simulink model "saturn_thermal4"  (R2021a)
settings: Solver=ode23t  StartTime=0.0  StopTime=80000  MaxStep=1000  RelTol=1e-3
values from neighbouring files (symbols this model uses):
  Ab = L*l    [Data_ini_thermal_analysis4.m]    (also in Data_ini_thermal_analysis5.m)
  As = l*l    [Data_ini_thermal_analysis4.m]    (also in Data_ini_thermal_analysis5.m)
  D_st = 1224526    [Data_ini_thermal_analysis4.m]    (also in Data_ini_thermal_analysis5.m)
  ecc_sc = 0    [Data_ini_thermal_analysis4.m]    (also in Data_ini_thermal_analysis5.m)
  ecc_t = 0.0293    [Data_ini_thermal_analysis4.m]    (also in Data_ini_thermal_analysis5.m)
  incl_ax_s = deg2rad(26.73)    [Data_ini_thermal_analysis4.m]    (also in Data_ini_thermal_analysis5.m)
  incl_sc = deg2rad(90+45)    [Data_ini_thermal_analysis4.m]    (also in Data_ini_thermal_analysis5.m)
  incl_t = deg2rad(0.3485)    [Data_ini_thermal_analysis4.m]    (also in Data_ini_thermal_analysis5.m)
  mean_motion_sc = 2*pi/period_sc    [Data_ini_thermal_analysis4.m]    (also in Data_ini_thermal_analysis5.m)
  mean_motion_t = (2*pi)/period_t    (= 4.56068561416e-06)    [Data_ini_thermal_analysis4.m]    (also in Data_ini_thermal_analysis5.m)
  mean_r_s = 1.427*10^9    (= 1427000000)    [Data_ini_thermal_analysis4.m]    (also in Data_ini_thermal_analysis5.m)
  mu_s = 37931187    [Data_ini_thermal_analysis4.m]    (also in Data_ini_thermal_analysis5.m)
  mu_t = 8971.15    [Data_ini_thermal_analysis4.m]    (also in Data_ini_thermal_analysis5.m)
  period_s = 29.45*365*24*3600    (= 928735200)    [Data_ini_thermal_analysis4.m]    (also in Data_ini_thermal_analysis5.m)
  period_t = 15.945421*24*3600    (= 1377684.3744)    [Data_ini_thermal_analysis4.m]    (also in Data_ini_thermal_analysis5.m)
  R_s = diam_s/2    (= 60268)    [Data_ini_thermal_analysis4.m]    (also in Data_ini_thermal_analysis5.m)
  R_t = 2576    [Data_ini_thermal_analysis4.m]    (also in Data_ini_thermal_analysis5.m)
  semajax_sc = 1500+R_t    (= 4076)    [Data_ini_thermal_analysis4.m]    (also in Data_ini_thermal_analysis5.m)
  semajax_t = 1221830    [Data_ini_thermal_analysis4.m]    (also in Data_ini_thermal_analysis5.m)
libraries: fl_lib x283, nesl_utility x27
(part 2 of 3)

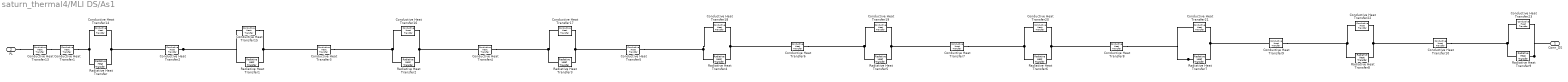
== system saturn_thermal4/MLI DS/As1 ==
  Conductive Heat Transfer{1..10} (10 alike) : fl_lib/Thermal/Thermal Elements/Conductive Heat Transfer  area=As m^2  thickness=s_kap m  th_cond=k_kap W/(m*K)  T_specify=off  T_priority=None  T=0 K  T_nominal_specify=off  T_nominal_unit=K  T_nominal_value=1  Q_specify=off  Q_priority=None  Q=0 W  Q_nominal_specify=off  Q_nominal_unit=W  Q_nominal_value=1
  Conductive Heat Transfer13 : fl_lib/Thermal/Thermal Elements/Conductive Heat Transfer  area=As m^2  thickness=s_al m  th_cond=k_al W/(m*K)  T_specify=off  T_priority=None  T=0 K  T_nominal_specify=off  T_nominal_unit=K  T_nominal_value=1  Q_specify=off  Q_priority=None  Q=0 W  Q_nominal_specify=off  Q_nominal_unit=W  Q_nominal_value=1
  Conductive Heat Transfer{14..23} (10 alike) : fl_lib/Thermal/Thermal Elements/Conductive Heat Transfer  area=A_net_new m^2  thickness=s_tfe_out m  th_cond=k_tfe W/(m*K)  T_specify=off  T_priority=None  T=0 K  T_nominal_specify=off  T_nominal_unit=K  T_nominal_value=1  Q_specify=off  Q_priority=None  Q=0 W  Q_nominal_specify=off  Q_nominal_unit=W  Q_nominal_value=1
  Radiative Heat Transfer{,1..9} (10 alike) : fl_lib/Thermal/Thermal Elements/Radiative Heat Transfer  area=A_empty m^2  rad_tr_coeff=Gr_kap_mli W/(m^2*K^4)  T_specify=off  T_priority=None  T=0 K  T_nominal_specify=off  T_nominal_unit=K  T_nominal_value=1  Q_specify=off  Q_priority=None  Q=0 W  Q_nominal_specify=off  Q_nominal_unit=W  Q_nominal_value=1
      settings: SourceProductBaseCode=SS  InternalSimscapePortConfiguration="{\"Bottom\":[],\"Left\":[{\"id\":\"A\",\"label\":\"A\",\"type\":\"foundation.thermal.thermal\"}],\"Right\":[{\"id\":\"B\",\"label\":\"B\",\"type\":\"foundation.thermal.thermal\"}],\"Top\":[]}"
  Conn_DS : PMIOPort  Side=Right
  PL : PMIOPort  Port=2  Side=Left
  connections:
  Radiative Heat Transfer/LConn1 -- Conductive Heat Transfer14/LConn1 -- Conductive Heat Transfer1/RConn1
  PL/RConn1 -- Conductive Heat Transfer13/LConn1
  Conductive Heat Transfer10/LConn1 -- Conductive Heat Transfer22/RConn1 -- Radiative Heat Transfer8/RConn1
  Conductive Heat Transfer9/RConn1 -- Conductive Heat Transfer22/LConn1 -- Radiative Heat Transfer8/LConn1
  Conductive Heat Transfer2/RConn1 -- Radiative Heat Transfer1/LConn1 -- Conductive Heat Transfer15/LConn1
  Radiative Heat Transfer9/RConn1 -- Conn_DS/RConn1 -- Conductive Heat Transfer23/RConn1
  Conductive Heat Transfer3/LConn1 -- Conductive Heat Transfer15/RConn1 -- Radiative Heat Transfer1/RConn1
  Conductive Heat Transfer4/LConn1 -- Conductive Heat Transfer16/RConn1 -- Radiative Heat Transfer2/RConn1
  Conductive Heat Transfer3/RConn1 -- Conductive Heat Transfer16/LConn1 -- Radiative Heat Transfer2/LConn1
  Conductive Heat Transfer2/LConn1 -- Radiative Heat Transfer/RConn1 -- Conductive Heat Transfer14/RConn1
  Conductive Heat Transfer10/RConn1 -- Conductive Heat Transfer23/LConn1 -- Radiative Heat Transfer9/LConn1
  Conductive Heat Transfer5/LConn1 -- Conductive Heat Transfer17/RConn1 -- Radiative Heat Transfer3/RConn1
  Conductive Heat Transfer6/LConn1 -- Conductive Heat Transfer18/RConn1 -- Radiative Heat Transfer4/RConn1
  Conductive Heat Transfer9/LConn1 -- Conductive Heat Transfer21/RConn1 -- Radiative Heat Transfer7/RConn1
  Conductive Heat Transfer7/RConn1 -- Conductive Heat Transfer20/LConn1 -- Radiative Heat Transfer6/LConn1
  Conductive Heat Transfer5/RConn1 -- Conductive Heat Transfer18/LConn1 -- Radiative Heat Transfer4/LConn1
  Conductive Heat Transfer13/RConn1 -- Conductive Heat Transfer1/LConn1
  Conductive Heat Transfer7/LConn1 -- Conductive Heat Transfer19/RConn1 -- Radiative Heat Transfer5/RConn1
  Conductive Heat Transfer4/RConn1 -- Radiative Heat Transfer3/LConn1 -- Conductive Heat Transfer17/LConn1
  Radiative Heat Transfer7/LConn1 -- Conductive Heat Transfer8/RConn1 -- Conductive Heat Transfer21/LConn1
  Conductive Heat Transfer8/LConn1 -- Conductive Heat Transfer20/RConn1 -- Radiative Heat Transfer6/RConn1
  Conductive Heat Transfer6/RConn1 -- Conductive Heat Transfer19/LConn1 -- Radiative Heat Transfer5/LConn1

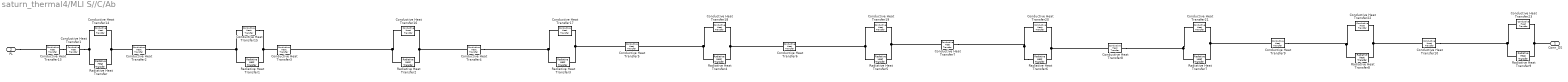
== system saturn_thermal4/MLI S//C/Ab ==
  Conductive Heat Transfer{1..10} (10 alike) : fl_lib/Thermal/Thermal Elements/Conductive Heat Transfer  area=Ab m^2  thickness=s_kap m  th_cond=k_kap W/(m*K)  T_specify=off  T_priority=None  T=0 K  T_nominal_specify=off  T_nominal_unit=K  T_nominal_value=1  Q_specify=off  Q_priority=None  Q=0 W  Q_nominal_specify=off  Q_nominal_unit=W  Q_nominal_value=1
  Conductive Heat Transfer13 : fl_lib/Thermal/Thermal Elements/Conductive Heat Transfer  area=Ab m^2  thickness=s_al m  th_cond=k_al W/(m*K)  T_specify=off  T_priority=None  T=0 K  T_nominal_specify=off  T_nominal_unit=K  T_nominal_value=1  Q_specify=off  Q_priority=None  Q=0 W  Q_nominal_specify=off  Q_nominal_unit=W  Q_nominal_value=1
  Conductive Heat Transfer{14..23} (10 alike) : fl_lib/Thermal/Thermal Elements/Conductive Heat Transfer  area=A_net_new_b m^2  thickness=s_tfe_out m  th_cond=k_tfe W/(m*K)  T_specify=off  T_priority=None  T=0 K  T_nominal_specify=off  T_nominal_unit=K  T_nominal_value=1  Q_specify=off  Q_priority=None  Q=0 W  Q_nominal_specify=off  Q_nominal_unit=W  Q_nominal_value=1
  Radiative Heat Transfer{,1..9} (10 alike) : fl_lib/Thermal/Thermal Elements/Radiative Heat Transfer  area=A_empty_b m^2  rad_tr_coeff=Gr_kap_mli W/(m^2*K^4)  T_specify=off  T_priority=None  T=0 K  T_nominal_specify=off  T_nominal_unit=K  T_nominal_value=1  Q_specify=off  Q_priority=None  Q=0 W  Q_nominal_specify=off  Q_nominal_unit=W  Q_nominal_value=1
      settings: SourceProductBaseCode=SS  InternalSimscapePortConfiguration="{\"Bottom\":[],\"Left\":[{\"id\":\"A\",\"label\":\"A\",\"type\":\"foundation.thermal.thermal\"}],\"Right\":[{\"id\":\"B\",\"label\":\"B\",\"type\":\"foundation.thermal.thermal\"}],\"Top\":[]}"
  Conn_DS : PMIOPort  Side=Right
  PL : PMIOPort  Port=2  Side=Left
  connections:
  Conductive Heat Transfer13/RConn1 -- Conductive Heat Transfer1/LConn1
  PL/RConn1 -- Conductive Heat Transfer13/LConn1
  Conductive Heat Transfer10/LConn1 -- Conductive Heat Transfer22/RConn1 -- Radiative Heat Transfer8/RConn1
  Conductive Heat Transfer9/RConn1 -- Conductive Heat Transfer22/LConn1 -- Radiative Heat Transfer8/LConn1
  Conductive Heat Transfer2/RConn1 -- Radiative Heat Transfer1/LConn1 -- Conductive Heat Transfer15/LConn1
  Conn_DS/RConn1 -- Conductive Heat Transfer23/RConn1 -- Radiative Heat Transfer9/RConn1
  Radiative Heat Transfer1/RConn1 -- Conductive Heat Transfer15/RConn1 -- Conductive Heat Transfer3/LConn1
  Conductive Heat Transfer4/LConn1 -- Conductive Heat Transfer16/RConn1 -- Radiative Heat Transfer2/RConn1
  Conductive Heat Transfer3/RConn1 -- Conductive Heat Transfer16/LConn1 -- Radiative Heat Transfer2/LConn1
  Conductive Heat Transfer2/LConn1 -- Conductive Heat Transfer14/RConn1 -- Radiative Heat Transfer/RConn1
  Conductive Heat Transfer10/RConn1 -- Conductive Heat Transfer23/LConn1 -- Radiative Heat Transfer9/LConn1
  Radiative Heat Transfer3/RConn1 -- Conductive Heat Transfer17/RConn1 -- Conductive Heat Transfer5/LConn1
  Conductive Heat Transfer6/LConn1 -- Radiative Heat Transfer4/RConn1 -- Conductive Heat Transfer18/RConn1
  Radiative Heat Transfer7/RConn1 -- Conductive Heat Transfer21/RConn1 -- Conductive Heat Transfer9/LConn1
  Radiative Heat Transfer6/LConn1 -- Conductive Heat Transfer20/LConn1 -- Conductive Heat Transfer7/RConn1
  Conductive Heat Transfer5/RConn1 -- Conductive Heat Transfer18/LConn1 -- Radiative Heat Transfer4/LConn1
  Conductive Heat Transfer14/LConn1 -- Conductive Heat Transfer1/RConn1 -- Radiative Heat Transfer/LConn1
  Conductive Heat Transfer7/LConn1 -- Conductive Heat Transfer19/RConn1 -- Radiative Heat Transfer5/RConn1
  Conductive Heat Transfer4/RConn1 -- Radiative Heat Transfer3/LConn1 -- Conductive Heat Transfer17/LConn1
  Conductive Heat Transfer8/RConn1 -- Radiative Heat Transfer7/LConn1 -- Conductive Heat Transfer21/LConn1
  Conductive Heat Transfer8/LConn1 -- Radiative Heat Transfer6/RConn1 -- Conductive Heat Transfer20/RConn1
  Conductive Heat Transfer6/RConn1 -- Radiative Heat Transfer5/LConn1 -- Conductive Heat Transfer19/LConn1

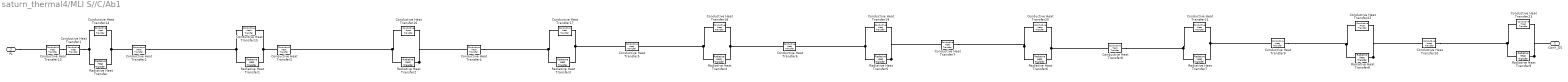
== system saturn_thermal4/MLI S//C/Ab1 ==
  Conductive Heat Transfer{1..10} (10 alike) : fl_lib/Thermal/Thermal Elements/Conductive Heat Transfer  area=Ab m^2  thickness=s_kap m  th_cond=k_kap W/(m*K)  T_specify=off  T_priority=None  T=0 K  T_nominal_specify=off  T_nominal_unit=K  T_nominal_value=1  Q_specify=off  Q_priority=None  Q=0 W  Q_nominal_specify=off  Q_nominal_unit=W  Q_nominal_value=1
  Conductive Heat Transfer13 : fl_lib/Thermal/Thermal Elements/Conductive Heat Transfer  area=Ab m^2  thickness=s_al m  th_cond=k_al W/(m*K)  T_specify=off  T_priority=None  T=0 K  T_nominal_specify=off  T_nominal_unit=K  T_nominal_value=1  Q_specify=off  Q_priority=None  Q=0 W  Q_nominal_specify=off  Q_nominal_unit=W  Q_nominal_value=1
  Conductive Heat Transfer{14..23} (10 alike) : fl_lib/Thermal/Thermal Elements/Conductive Heat Transfer  area=A_net_new_b m^2  thickness=s_tfe_out m  th_cond=k_tfe W/(m*K)  T_specify=off  T_priority=None  T=0 K  T_nominal_specify=off  T_nominal_unit=K  T_nominal_value=1  Q_specify=off  Q_priority=None  Q=0 W  Q_nominal_specify=off  Q_nominal_unit=W  Q_nominal_value=1
  Radiative Heat Transfer{,1..9} (10 alike) : fl_lib/Thermal/Thermal Elements/Radiative Heat Transfer  area=A_empty_b m^2  rad_tr_coeff=Gr_kap_mli W/(m^2*K^4)  T_specify=off  T_priority=None  T=0 K  T_nominal_specify=off  T_nominal_unit=K  T_nominal_value=1  Q_specify=off  Q_priority=None  Q=0 W  Q_nominal_specify=off  Q_nominal_unit=W  Q_nominal_value=1
      settings: SourceProductBaseCode=SS  InternalSimscapePortConfiguration="{\"Bottom\":[],\"Left\":[{\"id\":\"A\",\"label\":\"A\",\"type\":\"foundation.thermal.thermal\"}],\"Right\":[{\"id\":\"B\",\"label\":\"B\",\"type\":\"foundation.thermal.thermal\"}],\"Top\":[]}"
  Conn_DS : PMIOPort  Side=Right
  PL : PMIOPort  Port=2  Side=Left
  connections:
  Conductive Heat Transfer19/LConn1 -- Radiative Heat Transfer5/LConn1 -- Conductive Heat Transfer6/RConn1
  Conductive Heat Transfer20/RConn1 -- Radiative Heat Transfer6/RConn1 -- Conductive Heat Transfer8/LConn1
  Conductive Heat Transfer21/LConn1 -- Radiative Heat Transfer7/LConn1 -- Conductive Heat Transfer8/RConn1
  Conductive Heat Transfer17/LConn1 -- Radiative Heat Transfer3/LConn1 -- Conductive Heat Transfer4/RConn1
  Radiative Heat Transfer5/RConn1 -- Conductive Heat Transfer19/RConn1 -- Conductive Heat Transfer7/LConn1
  Radiative Heat Transfer/LConn1 -- Conductive Heat Transfer1/RConn1 -- Conductive Heat Transfer14/LConn1
  Radiative Heat Transfer4/LConn1 -- Conductive Heat Transfer18/LConn1 -- Conductive Heat Transfer5/RConn1
  Conductive Heat Transfer7/RConn1 -- Conductive Heat Transfer20/LConn1 -- Radiative Heat Transfer6/LConn1
  Conductive Heat Transfer9/LConn1 -- Conductive Heat Transfer21/RConn1 -- Radiative Heat Transfer7/RConn1
  Conductive Heat Transfer18/RConn1 -- Radiative Heat Transfer4/RConn1 -- Conductive Heat Transfer6/LConn1
  Conductive Heat Transfer5/LConn1 -- Conductive Heat Transfer17/RConn1 -- Radiative Heat Transfer3/RConn1
  Radiative Heat Transfer9/LConn1 -- Conductive Heat Transfer23/LConn1 -- Conductive Heat Transfer10/RConn1
  Radiative Heat Transfer/RConn1 -- Conductive Heat Transfer14/RConn1 -- Conductive Heat Transfer2/LConn1
  Radiative Heat Transfer2/LConn1 -- Conductive Heat Transfer16/LConn1 -- Conductive Heat Transfer3/RConn1
  Radiative Heat Transfer2/RConn1 -- Conductive Heat Transfer16/RConn1 -- Conductive Heat Transfer4/LConn1
  Conductive Heat Transfer3/LConn1 -- Conductive Heat Transfer15/RConn1 -- Radiative Heat Transfer1/RConn1
  Radiative Heat Transfer9/RConn1 -- Conductive Heat Transfer23/RConn1 -- Conn_DS/RConn1
  Conductive Heat Transfer15/LConn1 -- Radiative Heat Transfer1/LConn1 -- Conductive Heat Transfer2/RConn1
  Radiative Heat Transfer8/LConn1 -- Conductive Heat Transfer22/LConn1 -- Conductive Heat Transfer9/RConn1
  Radiative Heat Transfer8/RConn1 -- Conductive Heat Transfer22/RConn1 -- Conductive Heat Transfer10/LConn1
  PL/RConn1 -- Conductive Heat Transfer13/LConn1
  Conductive Heat Transfer13/RConn1 -- Conductive Heat Transfer1/LConn1

== system saturn_thermal4/active heat control box/Subsystem ==
  signal : Inport
  reference : Inport  Port=2
  on case : Inport  Port=3
  off case : Inport  Port=4
  Controlled Heat Flow Rate Source : fl_lib/Thermal/Thermal Sources/Controlled Heat Flow Rate Source
  Data Type Conversion : DataTypeConversion  OutDataTypeStr=double
  Relational Operator : RelationalOperator  Operator=<=  OutDataTypeStr=boolean  RndMeth=Simplest
  Simulink-PS Converter : nesl_utility/Simulink-PS Converter  PhysicalDomain=network_engine_domain  SubClassName=ps_input  LeftPortType=input  RightPortType=output  PseudoPeriodic=off  Frequencies=[]  NoiseDistribution=none  NoiseParameters=[]  Unit=1  AffineConversion=off  FilteringAndDerivatives=provide  SimscapeFilterOrder=1  InputFilterTimeConstant=0.001  UdotUserProvided=0
      settings: SourceProductBaseCode=PW,SS
  Switch : Switch  Criteria=u2 > Threshold
  Thermal Reference1 : fl_lib/Thermal/Thermal Elements/Thermal Reference
  heat block : PMIOPort  Side=Right
  Output : Outport
  wires:
  Data Type Conversion/1 -> Simulink-PS Converter/1
  signal/1 -> Relational Operator/1
  off case/1 -> Switch/3
  Relational Operator/1 -> Output/1, Switch/2
  Switch/1 -> Data Type Conversion/1
  reference/1 -> Relational Operator/2
  on case/1 -> Switch/1
  connections:
  Thermal Reference1/LConn1 -- Controlled Heat Flow Rate Source/RConn2
  Controlled Heat Flow Rate Source/LConn1 -- heat block/RConn1
  Simulink-PS Converter/RConn1 -- Controlled Heat Flow Rate Source/RConn1

== system saturn_thermal4/active heat control box/Subsystem1 ==
  signal : Inport
  reference : Inport  Port=2
  off case : Inport  Port=3
  Conductive Heat Transfer1 : fl_lib/Thermal/Thermal Elements/Conductive Heat Transfer  area=As m^2  thickness=0.3 m  th_cond=k_al W/(m*K)  T_specify=off  T_priority=None  T=0 K  T_nominal_specify=off  T_nominal_unit=K  T_nominal_value=1  Q_specify=off  Q_priority=None  Q=0 W  Q_nominal_specify=off  Q_nominal_unit=W  Q_nominal_value=1
  Controlled Temperature Source : fl_lib/Thermal/Thermal Sources/Controlled Temperature Source
  Data Type Conversion : DataTypeConversion  OutDataTypeStr=double
  Deep space1 : fl_lib/Thermal/Thermal Sources/Temperature Source  temperature=T_ds K
  PS-Simulink Converter : nesl_utility/PS-Simulink Converter  PhysicalDomain=network_engine_domain  SubClassName=ps_output  LeftPortType=input  RightPortType=output  PseudoPeriodic=off  Frequencies=[]  Unit=inherit  AffineConversion=off
      settings: SourceProductBaseCode=PW,SS
  Radiative Heat Transfer3 : fl_lib/Thermal/Thermal Elements/Radiative Heat Transfer  area=5*As m^2  rad_tr_coeff=Gr_al W/(m^2*K^4)  T_specify=off  T_priority=None  T=0 K  T_nominal_specify=off  T_nominal_unit=K  T_nominal_value=1  Q_specify=off  Q_priority=None  Q=0 W  Q_nominal_specify=off  Q_nominal_unit=W  Q_nominal_value=1
      settings: SourceProductBaseCode=SS  InternalSimscapePortConfiguration="{\"Bottom\":[],\"Left\":[{\"id\":\"A\",\"label\":\"A\",\"type\":\"foundation.thermal.thermal\"}],\"Right\":[{\"id\":\"B\",\"label\":\"B\",\"type\":\"foundation.thermal.thermal\"}],\"Top\":[]}"
  Radiator : fl_lib/Thermal/Thermal Elements/Thermal Mass  mass=m_rad kg  sp_heat=cp_al J/kg/K  T_specify=on  T_priority=High  T=3 K  T_nominal_specify=off  T_nominal_unit=K  T_nominal_value=1  Q_specify=off  Q_priority=None  Q=0 W  Q_nominal_specify=off  Q_nominal_unit=W  Q_nominal_value=1
  Relational Operator : RelationalOperator  OutDataTypeStr=boolean  RndMeth=Simplest
  Simulink-PS Converter : nesl_utility/Simulink-PS Converter  PhysicalDomain=network_engine_domain  SubClassName=ps_input  LeftPortType=input  RightPortType=output  PseudoPeriodic=off  Frequencies=[]  NoiseDistribution=none  NoiseParameters=[]  Unit=1  AffineConversion=off  FilteringAndDerivatives=provide  SimscapeFilterOrder=1  InputFilterTimeConstant=0.001  UdotUserProvided=0
      settings: SourceProductBaseCode=PW,SS
  Solver Configuration : nesl_utility/Solver Configuration  PhysicalDomain=network_engine_domain  SubClassName=solver  LeftPortType=input  RightPortType=generic  Tones=[]  Harmonics=[]  SimulateNoise=off  Profile=off  UseLocalSampling=off  EnableSwitchedLinearOptims=on  FrequencyDomain=off  UseCCode=off  RelTol=0.001  AbsTol=1e-06  MinStep=1e-09  ToWorkspace=off  RevertToSquareIcSolve=off  NumHomotopyIterations=100  PhasorMode=off  PhasorModeNumHarmonics=1  DoDC=off  ResidualTolerance=1e-09  UseLocalSolver=off  LocalSolverChoice=NE_BACKWARD_EULER_ADVANCER  LocalSolverSampleTime=0.001  DoFixedCost=off  MaxNonlinIter=3  MaxModeIter=2  ComputeImpulses=off  ImpulseIterations=2  LinearAlgebra=auto  EquationFormulation=NE_TIME_EF  DelaysMemoryBudget=1024  AutomaticFiltering=on  FilteringTimeConstant=0.001  PartitionStorageMethod=AS_NEEDED  PartitionMemoryBudget=1024  PartitionMethod=ROBUST
      settings: SourceProductBaseCode=PW,SS
  Switch : Switch  Criteria=u2 > Threshold
  Temperature Sensor : fl_lib/Thermal/Thermal Sensors/Temperature Sensor
  Thermal Reference1 : fl_lib/Thermal/Thermal Elements/Thermal Reference
  Thermal Reference2 : fl_lib/Thermal/Thermal Elements/Thermal Reference
  heat block : PMIOPort  Side=Left
  Output : Outport
  wires:
  reference/1 -> Relational Operator/2
  Switch/1 -> Data Type Conversion/1
  Relational Operator/1 -> Output/1, Switch/2
  off case/1 -> Switch/3
  signal/1 -> Relational Operator/1
  Data Type Conversion/1 -> Simulink-PS Converter/1
  PS-Simulink Converter/1 -> Switch/1
  connections:
  Simulink-PS Converter/RConn1 -- Controlled Temperature Source/RConn1
  Solver Configuration/RConn1 -- Thermal Reference1/LConn1 -- Controlled Temperature Source/RConn2
  heat block/RConn1 -- Temperature Sensor/LConn1
  Temperature Sensor/RConn2 -- PS-Simulink Converter/LConn1
  Temperature Sensor/RConn1 -- Thermal Reference2/LConn1
  Conductive Heat Transfer1/RConn1 -- Radiative Heat Transfer3/LConn1 -- Radiator/LConn1
  Controlled Temperature Source/LConn1 -- Conductive Heat Transfer1/LConn1
  Radiative Heat Transfer3/RConn1 -- Deep space1/LConn1

== system saturn_thermal4/active heat control ref + antenna/Subsystem ==
  signal : Inport
  reference : Inport  Port=2
  on case : Inport  Port=3
  off case : Inport  Port=4
  Controlled Heat Flow Rate Source : fl_lib/Thermal/Thermal Sources/Controlled Heat Flow Rate Source
  Data Type Conversion : DataTypeConversion  OutDataTypeStr=double
  Relational Operator : RelationalOperator  Operator=<=  OutDataTypeStr=boolean  RndMeth=Simplest
  Simulink-PS Converter : nesl_utility/Simulink-PS Converter  PhysicalDomain=network_engine_domain  SubClassName=ps_input  LeftPortType=input  RightPortType=output  PseudoPeriodic=off  Frequencies=[]  NoiseDistribution=none  NoiseParameters=[]  Unit=1  AffineConversion=off  FilteringAndDerivatives=provide  SimscapeFilterOrder=1  InputFilterTimeConstant=0.001  UdotUserProvided=0
      settings: SourceProductBaseCode=PW,SS
  Switch : Switch  Criteria=u2 > Threshold
  Thermal Reference1 : fl_lib/Thermal/Thermal Elements/Thermal Reference
  heat block : PMIOPort  Side=Right
  Output : Outport
  wires:
  Data Type Conversion/1 -> Simulink-PS Converter/1
  signal/1 -> Relational Operator/1
  off case/1 -> Switch/3
  Relational Operator/1 -> Output/1, Switch/2
  Switch/1 -> Data Type Conversion/1
  reference/1 -> Relational Operator/2
  on case/1 -> Switch/1
  connections:
  Thermal Reference1/LConn1 -- Controlled Heat Flow Rate Source/RConn2
  Controlled Heat Flow Rate Source/LConn1 -- heat block/RConn1
  Simulink-PS Converter/RConn1 -- Controlled Heat Flow Rate Source/RConn1

== system saturn_thermal4/active heat control ref + antenna/Subsystem1 ==
  signal : Inport
  reference : Inport  Port=2
  off case : Inport  Port=3
  Conductive Heat Transfer1 : fl_lib/Thermal/Thermal Elements/Conductive Heat Transfer  area=As m^2  thickness=0.3 m  th_cond=k_al W/(m*K)  T_specify=off  T_priority=None  T=0 K  T_nominal_specify=off  T_nominal_unit=K  T_nominal_value=1  Q_specify=off  Q_priority=None  Q=0 W  Q_nominal_specify=off  Q_nominal_unit=W  Q_nominal_value=1
  Controlled Temperature Source : fl_lib/Thermal/Thermal Sources/Controlled Temperature Source
  Data Type Conversion : DataTypeConversion  OutDataTypeStr=double
  Deep space1 : fl_lib/Thermal/Thermal Sources/Temperature Source  temperature=T_ds K
  PS-Simulink Converter : nesl_utility/PS-Simulink Converter  PhysicalDomain=network_engine_domain  SubClassName=ps_output  LeftPortType=input  RightPortType=output  PseudoPeriodic=off  Frequencies=[]  Unit=inherit  AffineConversion=off
      settings: SourceProductBaseCode=PW,SS
  Radiative Heat Transfer3 : fl_lib/Thermal/Thermal Elements/Radiative Heat Transfer  area=5*As m^2  rad_tr_coeff=Gr_al W/(m^2*K^4)  T_specify=off  T_priority=None  T=0 K  T_nominal_specify=off  T_nominal_unit=K  T_nominal_value=1  Q_specify=off  Q_priority=None  Q=0 W  Q_nominal_specify=off  Q_nominal_unit=W  Q_nominal_value=1
      settings: SourceProductBaseCode=SS  InternalSimscapePortConfiguration="{\"Bottom\":[],\"Left\":[{\"id\":\"A\",\"label\":\"A\",\"type\":\"foundation.thermal.thermal\"}],\"Right\":[{\"id\":\"B\",\"label\":\"B\",\"type\":\"foundation.thermal.thermal\"}],\"Top\":[]}"
  Radiator : fl_lib/Thermal/Thermal Elements/Thermal Mass  mass=m_rad kg  sp_heat=cp_al J/kg/K  T_specify=on  T_priority=High  T=3 K  T_nominal_specify=off  T_nominal_unit=K  T_nominal_value=1  Q_specify=off  Q_priority=None  Q=0 W  Q_nominal_specify=off  Q_nominal_unit=W  Q_nominal_value=1
  Relational Operator : RelationalOperator  OutDataTypeStr=boolean  RndMeth=Simplest
  Simulink-PS Converter : nesl_utility/Simulink-PS Converter  PhysicalDomain=network_engine_domain  SubClassName=ps_input  LeftPortType=input  RightPortType=output  PseudoPeriodic=off  Frequencies=[]  NoiseDistribution=none  NoiseParameters=[]  Unit=1  AffineConversion=off  FilteringAndDerivatives=provide  SimscapeFilterOrder=1  InputFilterTimeConstant=0.001  UdotUserProvided=0
      settings: SourceProductBaseCode=PW,SS
  Solver Configuration : nesl_utility/Solver Configuration  PhysicalDomain=network_engine_domain  SubClassName=solver  LeftPortType=input  RightPortType=generic  Tones=[]  Harmonics=[]  SimulateNoise=off  Profile=off  UseLocalSampling=off  EnableSwitchedLinearOptims=on  FrequencyDomain=off  UseCCode=off  RelTol=0.001  AbsTol=1e-06  MinStep=1e-09  ToWorkspace=off  RevertToSquareIcSolve=off  NumHomotopyIterations=100  PhasorMode=off  PhasorModeNumHarmonics=1  DoDC=off  ResidualTolerance=1e-09  UseLocalSolver=off  LocalSolverChoice=NE_BACKWARD_EULER_ADVANCER  LocalSolverSampleTime=0.001  DoFixedCost=off  MaxNonlinIter=3  MaxModeIter=2  ComputeImpulses=off  ImpulseIterations=2  LinearAlgebra=auto  EquationFormulation=NE_TIME_EF  DelaysMemoryBudget=1024  AutomaticFiltering=on  FilteringTimeConstant=0.001  PartitionStorageMethod=AS_NEEDED  PartitionMemoryBudget=1024  PartitionMethod=ROBUST
      settings: SourceProductBaseCode=PW,SS
  Switch : Switch  Criteria=u2 > Threshold
  Temperature Sensor : fl_lib/Thermal/Thermal Sensors/Temperature Sensor
  Thermal Reference1 : fl_lib/Thermal/Thermal Elements/Thermal Reference
  Thermal Reference2 : fl_lib/Thermal/Thermal Elements/Thermal Reference
  heat block : PMIOPort  Side=Left
  Output : Outport
  wires:
  reference/1 -> Relational Operator/2
  Switch/1 -> Data Type Conversion/1
  Relational Operator/1 -> Output/1, Switch/2
  off case/1 -> Switch/3
  signal/1 -> Relational Operator/1
  Data Type Conversion/1 -> Simulink-PS Converter/1
  PS-Simulink Converter/1 -> Switch/1
  connections:
  Simulink-PS Converter/RConn1 -- Controlled Temperature Source/RConn1
  Solver Configuration/RConn1 -- Thermal Reference1/LConn1 -- Controlled Temperature Source/RConn2
  heat block/RConn1 -- Temperature Sensor/LConn1
  Temperature Sensor/RConn2 -- PS-Simulink Converter/LConn1
  Temperature Sensor/RConn1 -- Thermal Reference2/LConn1
  Conductive Heat Transfer1/RConn1 -- Radiative Heat Transfer3/LConn1 -- Radiator/LConn1
  Controlled Temperature Source/LConn1 -- Conductive Heat Transfer1/LConn1
  Radiative Heat Transfer3/RConn1 -- Deep space1/LConn1

== system saturn_thermal4/active heat control ref + antenna1/Subsystem ==
  signal : Inport
  reference : Inport  Port=2
  on case : Inport  Port=3
  off case : Inport  Port=4
  Controlled Heat Flow Rate Source : fl_lib/Thermal/Thermal Sources/Controlled Heat Flow Rate Source
  Data Type Conversion : DataTypeConversion  OutDataTypeStr=double
  Relational Operator : RelationalOperator  Operator=<=  OutDataTypeStr=boolean  RndMeth=Simplest
  Simulink-PS Converter : nesl_utility/Simulink-PS Converter  PhysicalDomain=network_engine_domain  SubClassName=ps_input  LeftPortType=input  RightPortType=output  PseudoPeriodic=off  Frequencies=[]  NoiseDistribution=none  NoiseParameters=[]  Unit=1  AffineConversion=off  FilteringAndDerivatives=provide  SimscapeFilterOrder=1  InputFilterTimeConstant=0.001  UdotUserProvided=0
      settings: SourceProductBaseCode=PW,SS
  Switch : Switch  Criteria=u2 > Threshold
  Thermal Reference1 : fl_lib/Thermal/Thermal Elements/Thermal Reference
  heat block : PMIOPort  Side=Right
  Output : Outport
  wires:
  Data Type Conversion/1 -> Simulink-PS Converter/1
  signal/1 -> Relational Operator/1
  off case/1 -> Switch/3
  Relational Operator/1 -> Output/1, Switch/2
  Switch/1 -> Data Type Conversion/1
  reference/1 -> Relational Operator/2
  on case/1 -> Switch/1
  connections:
  Thermal Reference1/LConn1 -- Controlled Heat Flow Rate Source/RConn2
  Controlled Heat Flow Rate Source/LConn1 -- heat block/RConn1
  Simulink-PS Converter/RConn1 -- Controlled Heat Flow Rate Source/RConn1

== system saturn_thermal4/active heat control ref + antenna1/Subsystem1 ==
  signal : Inport
  reference : Inport  Port=2
  off case : Inport  Port=3
  Conductive Heat Transfer1 : fl_lib/Thermal/Thermal Elements/Conductive Heat Transfer  area=As m^2  thickness=0.3 m  th_cond=k_al W/(m*K)  T_specify=off  T_priority=None  T=0 K  T_nominal_specify=off  T_nominal_unit=K  T_nominal_value=1  Q_specify=off  Q_priority=None  Q=0 W  Q_nominal_specify=off  Q_nominal_unit=W  Q_nominal_value=1
  Controlled Temperature Source : fl_lib/Thermal/Thermal Sources/Controlled Temperature Source
  Data Type Conversion : DataTypeConversion  OutDataTypeStr=double
  Deep space1 : fl_lib/Thermal/Thermal Sources/Temperature Source  temperature=T_ds K
  PS-Simulink Converter : nesl_utility/PS-Simulink Converter  PhysicalDomain=network_engine_domain  SubClassName=ps_output  LeftPortType=input  RightPortType=output  PseudoPeriodic=off  Frequencies=[]  Unit=inherit  AffineConversion=off
      settings: SourceProductBaseCode=PW,SS
  Radiative Heat Transfer3 : fl_lib/Thermal/Thermal Elements/Radiative Heat Transfer  area=5*As m^2  rad_tr_coeff=Gr_al W/(m^2*K^4)  T_specify=off  T_priority=None  T=0 K  T_nominal_specify=off  T_nominal_unit=K  T_nominal_value=1  Q_specify=off  Q_priority=None  Q=0 W  Q_nominal_specify=off  Q_nominal_unit=W  Q_nominal_value=1
      settings: SourceProductBaseCode=SS  InternalSimscapePortConfiguration="{\"Bottom\":[],\"Left\":[{\"id\":\"A\",\"label\":\"A\",\"type\":\"foundation.thermal.thermal\"}],\"Right\":[{\"id\":\"B\",\"label\":\"B\",\"type\":\"foundation.thermal.thermal\"}],\"Top\":[]}"
  Radiator : fl_lib/Thermal/Thermal Elements/Thermal Mass  mass=m_rad kg  sp_heat=cp_al J/kg/K  T_specify=on  T_priority=High  T=3 K  T_nominal_specify=off  T_nominal_unit=K  T_nominal_value=1  Q_specify=off  Q_priority=None  Q=0 W  Q_nominal_specify=off  Q_nominal_unit=W  Q_nominal_value=1
  Relational Operator : RelationalOperator  OutDataTypeStr=boolean  RndMeth=Simplest
  Simulink-PS Converter : nesl_utility/Simulink-PS Converter  PhysicalDomain=network_engine_domain  SubClassName=ps_input  LeftPortType=input  RightPortType=output  PseudoPeriodic=off  Frequencies=[]  NoiseDistribution=none  NoiseParameters=[]  Unit=1  AffineConversion=off  FilteringAndDerivatives=provide  SimscapeFilterOrder=1  InputFilterTimeConstant=0.001  UdotUserProvided=0
      settings: SourceProductBaseCode=PW,SS
  Solver Configuration : nesl_utility/Solver Configuration  PhysicalDomain=network_engine_domain  SubClassName=solver  LeftPortType=input  RightPortType=generic  Tones=[]  Harmonics=[]  SimulateNoise=off  Profile=off  UseLocalSampling=off  EnableSwitchedLinearOptims=on  FrequencyDomain=off  UseCCode=off  RelTol=0.001  AbsTol=1e-06  MinStep=1e-09  ToWorkspace=off  RevertToSquareIcSolve=off  NumHomotopyIterations=100  PhasorMode=off  PhasorModeNumHarmonics=1  DoDC=off  ResidualTolerance=1e-09  UseLocalSolver=off  LocalSolverChoice=NE_BACKWARD_EULER_ADVANCER  LocalSolverSampleTime=0.001  DoFixedCost=off  MaxNonlinIter=3  MaxModeIter=2  ComputeImpulses=off  ImpulseIterations=2  LinearAlgebra=auto  EquationFormulation=NE_TIME_EF  DelaysMemoryBudget=1024  AutomaticFiltering=on  FilteringTimeConstant=0.001  PartitionStorageMethod=AS_NEEDED  PartitionMemoryBudget=1024  PartitionMethod=ROBUST
      settings: SourceProductBaseCode=PW,SS
  Switch : Switch  Criteria=u2 > Threshold
  Temperature Sensor : fl_lib/Thermal/Thermal Sensors/Temperature Sensor
  Thermal Reference1 : fl_lib/Thermal/Thermal Elements/Thermal Reference
  Thermal Reference2 : fl_lib/Thermal/Thermal Elements/Thermal Reference
  heat block : PMIOPort  Side=Left
  Output : Outport
  wires:
  reference/1 -> Relational Operator/2
  Switch/1 -> Data Type Conversion/1
  Relational Operator/1 -> Output/1, Switch/2
  off case/1 -> Switch/3
  signal/1 -> Relational Operator/1
  Data Type Conversion/1 -> Simulink-PS Converter/1
  PS-Simulink Converter/1 -> Switch/1
  connections:
  Simulink-PS Converter/RConn1 -- Controlled Temperature Source/RConn1
  Solver Configuration/RConn1 -- Thermal Reference1/LConn1 -- Controlled Temperature Source/RConn2
  heat block/RConn1 -- Temperature Sensor/LConn1
  Temperature Sensor/RConn2 -- PS-Simulink Converter/LConn1
  Temperature Sensor/RConn1 -- Thermal Reference2/LConn1
  Conductive Heat Transfer1/RConn1 -- Radiative Heat Transfer3/LConn1 -- Radiator/LConn1
  Controlled Temperature Source/LConn1 -- Conductive Heat Transfer1/LConn1
  Radiative Heat Transfer3/RConn1 -- Deep space1/LConn1

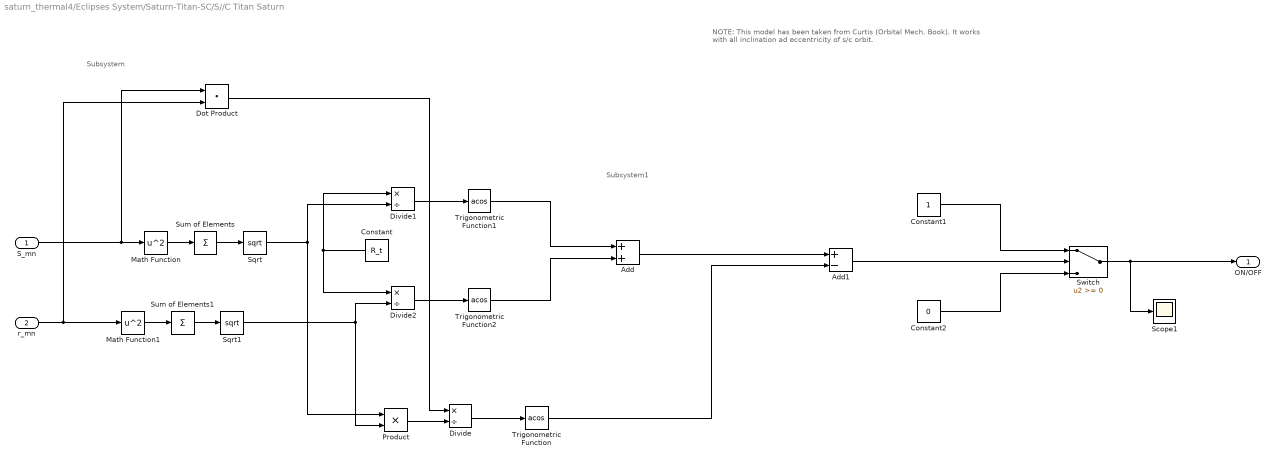
== system saturn_thermal4/Eclipses System/Saturn-Titan-SC/S//C Titan Saturn ==
  note: Subsystem
  note: Subsystem1
  note: NOTE: This model has been taken from Curtis (Orbital Mech. Book). It works with all inclination ad eccentricity of s/c orbit.
  S_mn : Inport
  r_mn : Inport  Port=2
  Add : Sum
  Add1 : Sum  Inputs=+-
  Constant : Constant  Value=R_t
  Constant1 : Constant
  Constant2 : Constant  Value=0
  Divide : Product  Inputs=*/
  Divide1 : Product  Inputs=*/
  Divide2 : Product  Inputs=*/
  Dot Product : DotProduct  InputSameDT=on  OutDataTypeStr=Inherit: Inherit via internal rule
  Math Function : Math  Operator=square  SaturateOnIntegerOverflow=on
  Math Function1 : Math  Operator=square  SaturateOnIntegerOverflow=on
  Product : Product
  Scope1 : Scope
  Sqrt : Sqrt  SaturateOnIntegerOverflow=on
  Sqrt1 : Sqrt  SaturateOnIntegerOverflow=on
  Sum of Elements : Sum  Inputs=+
  Sum of Elements1 : Sum  Inputs=+
  Switch : Switch
  Trigonometric Function : Trigonometry  Operator=acos
  Trigonometric Function1 : Trigonometry  Operator=acos
  Trigonometric Function2 : Trigonometry  Operator=acos
  ON/OFF : Outport
  wires:
  Add/1 -> Add1/1
  Add1/1 -> Switch/2
  Constant1/1 -> Switch/1
  Constant2/1 -> Switch/3
  Trigonometric Function1/1 -> Add/1
  Trigonometric Function2/1 -> Add/2
  Trigonometric Function/1 -> Add1/2
  Divide/1 -> Trigonometric Function/1
  Sum of Elements1/1 -> Sqrt1/1
  Constant/1 -> Divide2/1, Divide1/1
  S_mn/1 -> Dot Product/1, Math Function/1
  Sqrt1/1 -> Divide2/2, Product/2
  Product/1 -> Divide/2
  Sqrt/1 -> Divide1/2, Product/1
  Divide2/1 -> Trigonometric Function2/1
  Dot Product/1 -> Divide/1
  r_mn/1 -> Math Function1/1, Dot Product/2
  Math Function1/1 -> Sum of Elements1/1
  Divide1/1 -> Trigonometric Function1/1
  Math Function/1 -> Sum of Elements/1
  Sum of Elements/1 -> Sqrt/1
  Switch/1 -> ON/OFF/1, Scope1/1

== system saturn_thermal4/Eclipses System/Saturn-Titan-SC/S//C-Titan orbit ==
  Inertial Orbit Direction (Theta) : Subsystem
  Inertial Orbit Radius(Theta) : Subsystem
  Product : Product
  Subsystem : Subsystem
  True anomaly integration : Subsystem
  r_mn Scope : Scope
  r_mn : Outport
  wires:
  Product/1 -> r_mn Scope/1, r_mn/1  "r_mn"
  Inertial Orbit Direction (Theta)/1(r_vn) -> Product/2
  Inertial Orbit Radius(Theta)/1(r_mn) -> Subsystem/1(r_mn), Product/1
  True anomaly integration/1(Theta) -> Inertial Orbit Direction (Theta)/1(Theta), Inertial Orbit Radius(Theta)/1(Theta)  "Theta"

== system saturn_thermal4/Eclipses System/Saturn-Titan-SC/Titan-Saturn orbit ==
  Constant : Constant  Value=0
  Constant1 : Constant  Value=D_st
  Interpreted MATLAB Function : MATLABFcn  MATLABFcn=norm(u)
  Mux : Mux  Inputs=3
  Product : Product
  Product1 : Product
  Product2 : Product
  Scope : Scope
  Scope1 : Scope
  Subsystem : Subsystem
  Trigonometric Function : Trigonometry
  Trigonometric Function1 : Trigonometry  Operator=cos
  Trigonometric Function2 : Trigonometry
  Trigonometric Function3 : Trigonometry  Operator=cos
  Trigonometric Function4 : Trigonometry
  S_mn : Outport
  wires:
  Interpreted MATLAB Function/1 -> Scope1/1
  Product2/1 -> Scope/1, S_mn/1
  Mux/1 -> Product2/2, Interpreted MATLAB Function/1
  Constant1/1 -> Product2/1
  Trigonometric Function3/1 -> Product/2
  Trigonometric Function2/1 -> Product1/2
  Product/1 -> Mux/2
  Trigonometric Function4/1 -> Product1/1
  Trigonometric Function/1 -> Product/1
  Subsystem/1(theta_titan) -> Trigonometric Function2/1, Trigonometric Function/1, Trigonometric Function1/1
  Constant/1 -> Trigonometric Function3/1, Trigonometric Function4/1
  Trigonometric Function1/1 -> Mux/1
  Product1/1 -> Mux/3

== system saturn_thermal4/Eclipses System/Sun-Saturn-Titan/Saturn-Sun orbit ==
  Constant : Constant  Value=incl_ax_s
  Constant1 : Constant  Value=mean_r_s
  Interpreted MATLAB Function : MATLABFcn  MATLABFcn=norm(u)
  Mux : Mux  Inputs=3
  Product : Product
  Product1 : Product
  Product2 : Product
  Scope : Scope
  Scope1 : Scope
  Subsystem : Subsystem
  Trigonometric Function : Trigonometry
  Trigonometric Function1 : Trigonometry  Operator=cos
  Trigonometric Function2 : Trigonometry
  Trigonometric Function3 : Trigonometry  Operator=cos
  Trigonometric Function4 : Trigonometry
  S_mn : Outport
  wires:
  Product1/1 -> Mux/3
  Trigonometric Function1/1 -> Mux/1
  Constant/1 -> Trigonometric Function4/1, Trigonometric Function3/1
  Subsystem/1(theta_saturn) -> Trigonometric Function1/1, Trigonometric Function/1, Trigonometric Function2/1
  Trigonometric Function/1 -> Product/1
  Trigonometric Function4/1 -> Product1/1
  Product/1 -> Mux/2
  Trigonometric Function2/1 -> Product1/2
  Trigonometric Function3/1 -> Product/2
  Constant1/1 -> Product2/1
  Mux/1 -> Interpreted MATLAB Function/1, Product2/2
  Product2/1 -> S_mn/1, Scope/1
  Interpreted MATLAB Function/1 -> Scope1/1

== system saturn_thermal4/Eclipses System/Sun-Saturn-Titan/Titan-Saturn ==
  Inertial Orbit Direction (Theta) : Subsystem
  Inertial Orbit Radius(Theta) : Subsystem
  Product : Product
  Subsystem : Subsystem
  True anomaly integration : Subsystem
  r_mn Scope : Scope
  r_mn : Outport
  wires:
  True anomaly integration/1(Theta) -> Inertial Orbit Radius(Theta)/1(Theta), Inertial Orbit Direction (Theta)/1(Theta)  "Theta"
  Inertial Orbit Radius(Theta)/1(r_mn) -> Product/1, Subsystem/1(r_mn)
  Inertial Orbit Direction (Theta)/1(r_vn) -> Product/2
  Product/1 -> r_mn/1, r_mn Scope/1  "r_mn"

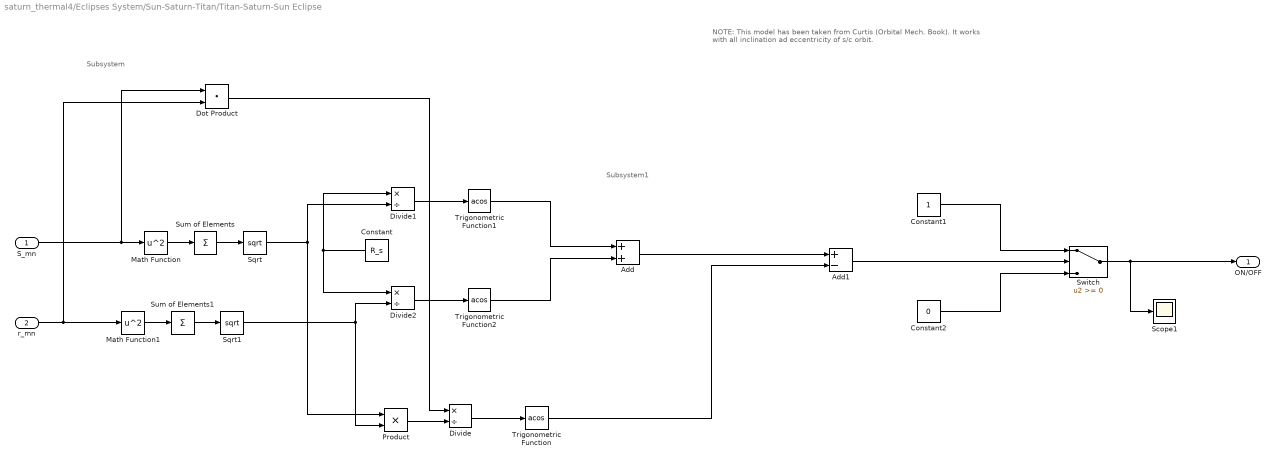
== system saturn_thermal4/Eclipses System/Sun-Saturn-Titan/Titan-Saturn-Sun Eclipse ==
  note: NOTE: This model has been taken from Curtis (Orbital Mech. Book). It works with all inclination ad eccentricity of s/c orbit.
  note: Subsystem1
  note: Subsystem
  S_mn : Inport
  r_mn : Inport  Port=2
  Add : Sum
  Add1 : Sum  Inputs=+-
  Constant : Constant  Value=R_s
  Constant1 : Constant
  Constant2 : Constant  Value=0
  Divide : Product  Inputs=*/
  Divide1 : Product  Inputs=*/
  Divide2 : Product  Inputs=*/
  Dot Product : DotProduct  InputSameDT=on  OutDataTypeStr=Inherit: Inherit via internal rule
  Math Function : Math  Operator=square  SaturateOnIntegerOverflow=on
  Math Function1 : Math  Operator=square  SaturateOnIntegerOverflow=on
  Product : Product
  Scope1 : Scope
  Sqrt : Sqrt  SaturateOnIntegerOverflow=on
  Sqrt1 : Sqrt  SaturateOnIntegerOverflow=on
  Sum of Elements : Sum  Inputs=+
  Sum of Elements1 : Sum  Inputs=+
  Switch : Switch
  Trigonometric Function : Trigonometry  Operator=acos
  Trigonometric Function1 : Trigonometry  Operator=acos
  Trigonometric Function2 : Trigonometry  Operator=acos
  ON/OFF : Outport
  wires:
  Switch/1 -> Scope1/1, ON/OFF/1
  Sum of Elements/1 -> Sqrt/1
  Math Function/1 -> Sum of Elements/1
  Divide1/1 -> Trigonometric Function1/1
  Math Function1/1 -> Sum of Elements1/1
  r_mn/1 -> Dot Product/2, Math Function1/1
  Dot Product/1 -> Divide/1
  Divide2/1 -> Trigonometric Function2/1
  Sqrt/1 -> Product/1, Divide1/2
  Product/1 -> Divide/2
  Sqrt1/1 -> Product/2, Divide2/2
  S_mn/1 -> Math Function/1, Dot Product/1
  Constant/1 -> Divide1/1, Divide2/1
  Sum of Elements1/1 -> Sqrt1/1
  Divide/1 -> Trigonometric Function/1
  Trigonometric Function/1 -> Add1/2
  Trigonometric Function2/1 -> Add/2
  Trigonometric Function1/1 -> Add/1
  Constant2/1 -> Switch/3
  Constant1/1 -> Switch/1
  Add1/1 -> Switch/2
  Add/1 -> Add1/1

== system saturn_thermal4/Eclipses System/Sun-Titan-SC/Ecliptic Orbital parameter1 ==
  Constant : Constant  Value=0
  Constant1 : Constant  Value=mean_r_s
  Interpreted MATLAB Function : MATLABFcn  MATLABFcn=norm(u)
  Mux : Mux  Inputs=3
  Product : Product
  Product1 : Product
  Product2 : Product
  Scope : Scope
  Scope1 : Scope
  Subsystem : Subsystem
  Trigonometric Function : Trigonometry
  Trigonometric Function1 : Trigonometry  Operator=cos
  Trigonometric Function2 : Trigonometry
  Trigonometric Function3 : Trigonometry  Operator=cos
  Trigonometric Function4 : Trigonometry
  S_mn : Outport
  wires:
  Interpreted MATLAB Function/1 -> Scope1/1
  Product2/1 -> Scope/1, S_mn/1
  Mux/1 -> Product2/2, Interpreted MATLAB Function/1
  Constant1/1 -> Product2/1
  Trigonometric Function3/1 -> Product/2
  Trigonometric Function2/1 -> Product1/2
  Product/1 -> Mux/2
  Trigonometric Function4/1 -> Product1/1
  Trigonometric Function/1 -> Product/1
  Subsystem/1(theta_sun) -> Trigonometric Function2/1, Trigonometric Function/1, Trigonometric Function1/1
  Constant/1 -> Trigonometric Function3/1, Trigonometric Function4/1
  Trigonometric Function1/1 -> Mux/1
  Product1/1 -> Mux/3

== system saturn_thermal4/Eclipses System/Sun-Titan-SC/Orbit Parameter1 ==
  Inertial Orbit Direction (Theta) : Subsystem
  Inertial Orbit Radius(Theta) : Subsystem
  Product : Product
  Subsystem : Subsystem
  True anomaly integration : Subsystem
  r_mn Scope : Scope
  r_mn : Outport
  wires:
  Product/1 -> r_mn Scope/1, r_mn/1  "r_mn"
  Inertial Orbit Direction (Theta)/1(r_vn) -> Product/2
  Inertial Orbit Radius(Theta)/1(r_mn) -> Subsystem/1(r_mn), Product/1
  True anomaly integration/1(Theta) -> Inertial Orbit Direction (Theta)/1(Theta), Inertial Orbit Radius(Theta)/1(Theta)  "Theta"

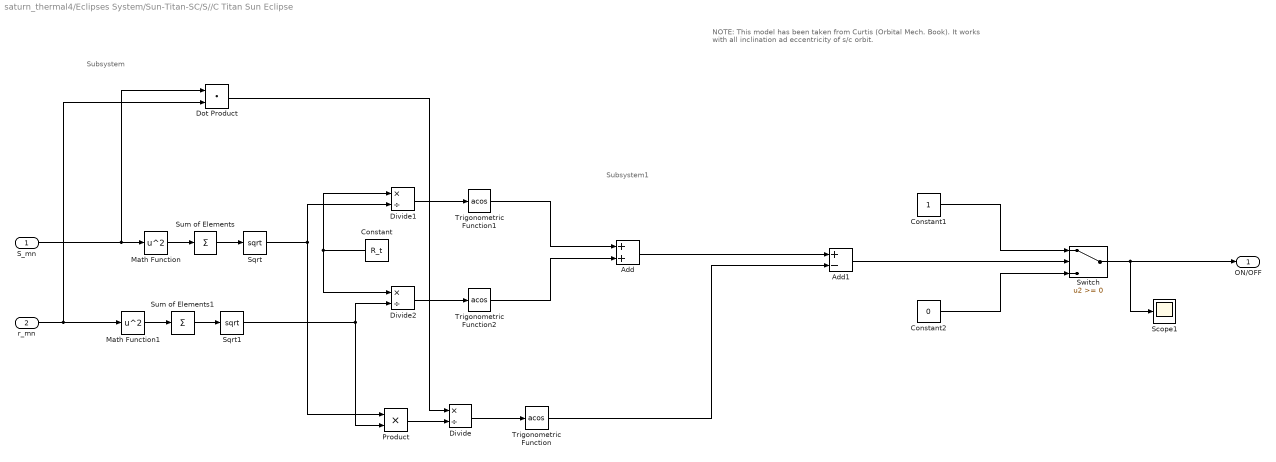
== system saturn_thermal4/Eclipses System/Sun-Titan-SC/S//C Titan Sun Eclipse ==
  note: Subsystem
  note: Subsystem1
  note: NOTE: This model has been taken from Curtis (Orbital Mech. Book). It works with all inclination ad eccentricity of s/c orbit.
  S_mn : Inport
  r_mn : Inport  Port=2
  Add : Sum
  Add1 : Sum  Inputs=+-
  Constant : Constant  Value=R_t
  Constant1 : Constant
  Constant2 : Constant  Value=0
  Divide : Product  Inputs=*/
  Divide1 : Product  Inputs=*/
  Divide2 : Product  Inputs=*/
  Dot Product : DotProduct  InputSameDT=on  OutDataTypeStr=Inherit: Inherit via internal rule
  Math Function : Math  Operator=square  SaturateOnIntegerOverflow=on
  Math Function1 : Math  Operator=square  SaturateOnIntegerOverflow=on
  Product : Product
  Scope1 : Scope
  Sqrt : Sqrt  SaturateOnIntegerOverflow=on
  Sqrt1 : Sqrt  SaturateOnIntegerOverflow=on
  Sum of Elements : Sum  Inputs=+
  Sum of Elements1 : Sum  Inputs=+
  Switch : Switch
  Trigonometric Function : Trigonometry  Operator=acos
  Trigonometric Function1 : Trigonometry  Operator=acos
  Trigonometric Function2 : Trigonometry  Operator=acos
  ON/OFF : Outport
  wires:
  Add/1 -> Add1/1
  Add1/1 -> Switch/2
  Constant1/1 -> Switch/1
  Constant2/1 -> Switch/3
  Trigonometric Function1/1 -> Add/1
  Trigonometric Function2/1 -> Add/2
  Trigonometric Function/1 -> Add1/2
  Divide/1 -> Trigonometric Function/1
  Sum of Elements1/1 -> Sqrt1/1
  Constant/1 -> Divide2/1, Divide1/1
  S_mn/1 -> Dot Product/1, Math Function/1
  Sqrt1/1 -> Divide2/2, Product/2
  Product/1 -> Divide/2
  Sqrt/1 -> Divide1/2, Product/1
  Divide2/1 -> Trigonometric Function2/1
  Dot Product/1 -> Divide/1
  r_mn/1 -> Math Function1/1, Dot Product/2
  Math Function1/1 -> Sum of Elements1/1
  Divide1/1 -> Trigonometric Function1/1
  Math Function/1 -> Sum of Elements/1
  Sum of Elements/1 -> Sqrt/1
  Switch/1 -> ON/OFF/1, Scope1/1

== system saturn_thermal4/Eclipses System/Saturn-Titan-SC/S//C-Titan orbit/Inertial Orbit Direction (Theta) ==
  note: definition of orbital path:
      |
      | cos(theta(t)) position wrt X_inertial (Gamma line for example)
      |
      | sin(theta(t))*cos(i) position wrt the Y_inertial
      |
      | sin(theta(t))*sin(i) position wrt the Z-inertial
      |
      | This vector define the s/c postition around the earth
  Theta : Inport
  Constant : Constant  Value=incl_sc
  Mux : Mux  Inputs=3
  Product : Product
  Product1 : Product
  Scope : Scope
  Trigonometric Function : Trigonometry
  Trigonometric Function1 : Trigonometry  Operator=cos
  Trigonometric Function2 : Trigonometry
  Trigonometric Function3 : Trigonometry  Operator=cos
  Trigonometric Function4 : Trigonometry
  r_vn : Outport
  wires:
  Mux/1 -> r_vn/1, Scope/1
  Trigonometric Function4/1 -> Product1/2
  Trigonometric Function2/1 -> Product1/1
  Trigonometric Function3/1 -> Product/2
  Trigonometric Function1/1 -> Mux/1
  Trigonometric Function/1 -> Product/1
  Constant/1 -> Trigonometric Function4/1, Trigonometric Function3/1
  Theta/1 -> Trigonometric Function2/1, Trigonometric Function/1, Trigonometric Function1/1
  Product1/1 -> Mux/3
  Product/1 -> Mux/2

== system saturn_thermal4/Eclipses System/Saturn-Titan-SC/S//C-Titan orbit/Inertial Orbit Radius(Theta) ==
  note: Orbital Radius magnitude computed as function of theta:
      |
      | R= a(1-ecc^2)/(1+ ecc*cos(theta(t))
  Theta : Inport
  Add : Sum
  Constant10 : Constant  Value=ecc_sc
  Constant3 : Constant  Value=semajax_sc
  Constant5 : Constant  Value=(1 - ecc_sc^2)
  Constant9 : Constant
  Divide1 : Product  Inputs=*/
  Product : Product
  Product1 : Product
  Trigonometric Function1 : Trigonometry  Operator=cos
  r_mn : Outport
  wires:
  Constant3/1 -> Product/1
  Constant10/1 -> Product1/1
  Theta/1 -> Trigonometric Function1/1
  Product/1 -> Divide1/1
  Constant5/1 -> Product/2
  Trigonometric Function1/1 -> Product1/2
  Constant9/1 -> Add/1
  Divide1/1 -> r_mn/1
  Add/1 -> Divide1/2
  Product1/1 -> Add/2

== system saturn_thermal4/Eclipses System/Saturn-Titan-SC/S//C-Titan orbit/Subsystem ==
  r_mn : Inport
  Add : Sum  Inputs=+-
  Constant1 : Constant  Value=mu_t
  Constant2 : Constant  Value=2
  Constant4 : Constant  Value=1/semajax_sc
  Divide : Product  Inputs=**
  Divide1 : Product  Inputs=*/
  Divide2 : Product  Inputs=*/
  Scope : Scope
  Scope1 : Scope
  Square Root : Sqrt  SaturateOnIntegerOverflow=on
  wires:
  Divide1/1 -> Scope1/1  "w_orb"
  Square Root/1 -> Scope/1, Divide1/1  "v_orb"
  r_mn/1 -> Divide2/2, Divide1/2
  Divide/1 -> Square Root/1
  Constant4/1 -> Add/2
  Divide2/1 -> Add/1
  Constant1/1 -> Divide/1
  Constant2/1 -> Divide2/1
  Add/1 -> Divide/2

== system saturn_thermal4/Eclipses System/Saturn-Titan-SC/S//C-Titan orbit/True anomaly integration ==
  Add1 : Sum
  Add2 : Sum  Inputs=+-
  Constant1 : Constant  Value=ecc_sc
  Constant7 : Constant
  Constant8 : Constant  Value=3/2
  Divide2 : Product  Inputs=*/
  Gain : Gain  Gain=ecc_sc
  Gain1 : Gain  Gain=mean_motion_sc
  Integrator : Integrator
  Math Function : Math  Operator=pow  SaturateOnIntegerOverflow=on
  Math Function1 : Math  Operator=square  SaturateOnIntegerOverflow=on
  Math Function2 : Math  Operator=square  SaturateOnIntegerOverflow=on
  Scope : Scope
  Trigonometric Function : Trigonometry  Operator=cos
  Theta : Outport
  wires:
  Add2/1 -> Math Function/1
  Math Function2/1 -> Add2/2
  Constant1/1 -> Math Function2/1
  Math Function1/1 -> Gain1/1
  Constant8/1 -> Math Function/2
  Gain1/1 -> Divide2/1
  Trigonometric Function/1 -> Gain/1
  Math Function/1 -> Divide2/2
  Add1/1 -> Math Function1/1
  Divide2/1 -> Integrator/1  "Theta_dot"
  Integrator/1 -> Theta/1, Scope/1, Trigonometric Function/1  "Theta"
  Constant7/1 -> Add2/1, Add1/2
  Gain/1 -> Add1/1

== system saturn_thermal4/Eclipses System/Saturn-Titan-SC/Titan-Saturn orbit/Subsystem ==
  note: Note: if the sun direction and the earth direction are parallel the Attitude Determinantion Algorithm wil stop to work due to sigularity value in the inertial frame direction (this matrix need to be invertible) so the theta sun integration must start with a value different from 0 or 180 deg. The alignament condition will arise again after a certain number of orbit periods (in 4 orbits this condition will not arise).
  Constant2 : Constant  Value=2*pi
  Constant3 : Constant  Value=period_t
  Divide : Product  Inputs=*/
  Integrator : Integrator
  Scope : Scope
  theta_titan : Outport
  wires:
  Integrator/1 -> Scope/1, theta_titan/1
  Divide/1 -> Integrator/1  "n_sun"
  Constant3/1 -> Divide/2
  Constant2/1 -> Divide/1

== system saturn_thermal4/Eclipses System/Sun-Saturn-Titan/Saturn-Sun orbit/Subsystem ==
  Constant2 : Constant  Value=2*pi
  Constant3 : Constant  Value=period_s
  Divide : Product  Inputs=*/
  Integrator : Integrator  InitialCondition=pi/2
  Scope : Scope
  theta_saturn : Outport
  wires:
  Constant2/1 -> Divide/1
  Constant3/1 -> Divide/2
  Divide/1 -> Integrator/1  "n_saturn"
  Integrator/1 -> theta_saturn/1, Scope/1

== system saturn_thermal4/Eclipses System/Sun-Saturn-Titan/Titan-Saturn/Inertial Orbit Direction (Theta) ==
  note: definition of orbital path:
      |
      | cos(theta(t)) position wrt X_inertial (Gamma line for example)
      |
      | sin(theta(t))*cos(i) position wrt the Y_inertial
      |
      | sin(theta(t))*sin(i) position wrt the Z-inertial
      |
      | This vector define the s/c postition around the earth
  Theta : Inport
  Constant : Constant  Value=incl_t
  Mux : Mux  Inputs=3
  Product : Product
  Product1 : Product
  Scope : Scope
  Trigonometric Function : Trigonometry
  Trigonometric Function1 : Trigonometry  Operator=cos
  Trigonometric Function2 : Trigonometry
  Trigonometric Function3 : Trigonometry  Operator=cos
  Trigonometric Function4 : Trigonometry
  r_vn : Outport
  wires:
  Product/1 -> Mux/2
  Product1/1 -> Mux/3
  Theta/1 -> Trigonometric Function1/1, Trigonometric Function/1, Trigonometric Function2/1
  Constant/1 -> Trigonometric Function3/1, Trigonometric Function4/1
  Trigonometric Function/1 -> Product/1
  Trigonometric Function1/1 -> Mux/1
  Trigonometric Function3/1 -> Product/2
  Trigonometric Function2/1 -> Product1/1
  Trigonometric Function4/1 -> Product1/2
  Mux/1 -> Scope/1, r_vn/1
